simulink model "hybridSysSim"  (R2014b)
settings: Solver=ode45  SolverMode=SingleTasking  StartTime=0.0  StopTime=5  RelTol=1e-3
(part 1 of 2)
settings Model: Creator=Ricardo  LastModifiedBy=ricardog
settings OptimizationCC: BlockReduction=off  BooleanDataType=off
settings DebuggingCC: SaveWithParameterizedLinksMsg=none  UnderspecifiedInitializationDetection=Classic  MergeDetectMultiDrivingBlocksExec=none  SignalResolutionControl=TryResolveAllWithWarning  SolverPrmCheckMsg=none
settings HardwareCC: TargetUnknown=on

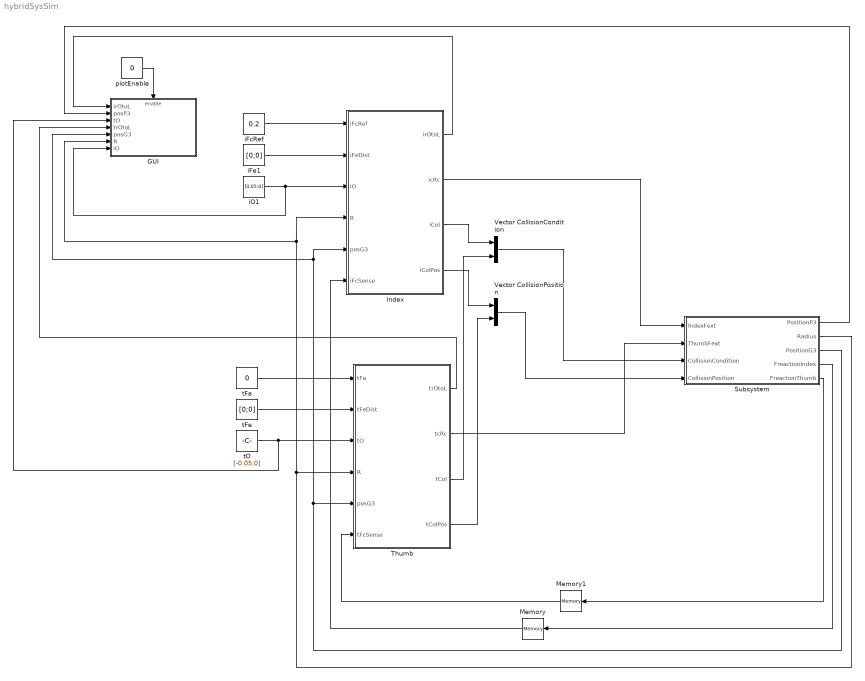
== system hybridSysSim ==
  GUI : Subsystem  TreatAsAtomicUnit=on
  Index : Subsystem
  Memory : Memory  InheritSampleTime=on
  Memory1 : Memory  InheritSampleTime=on
  Subsystem : Subsystem
  Thumb : Subsystem
  Vector CollisionCondition : Concatenate  Mode=Multidimensional array  ConcatenateDimension=2
  Vector CollisionPosition : Concatenate  Mode=Multidimensional array  ConcatenateDimension=2
  iFcRef : Constant  Value=0.2
  iFe1 : Constant  Value=[0;0]
  iO1 : Constant  Value=[0.05;0]
  plotEnable : Constant  Value=0
  tFa : Constant  Value=0
  tFe : Constant  Value=[0;0]
  tO : Constant  Value=[-0.05;0]
  wires:
  Thumb/2(tcRc) -> Subsystem/2(ThumbFext)
  plotEnable/1 -> GUI/Enable
  iFcRef/1 -> Index/1(iFcRef)
  iFe1/1 -> Index/2(iFeDist)
  iO1/1 -> GUI/7(iO), Index/3(iO)
  Index/3(iCol) -> Vector CollisionCondition/1
  Vector CollisionCondition/1 -> Subsystem/3(CollisionCondition)
  Vector CollisionPosition/1 -> Subsystem/4(CollisionPosition)
  Index/2(icRc) -> Subsystem/1(IndexFext)
  Subsystem/3(PositionG3) -> Thumb/5(posG3), GUI/5(posG3), Index/5(posG3)
  Subsystem/2(Radius) -> Thumb/4(R), GUI/6(R), Index/4(R)
  Subsystem/4(FreactionIndex) -> Memory/1
  Memory/1 -> Index/6(iFcSense)
  Index/4(iColPos) -> Vector CollisionPosition/1
  Index/1(irOtoL) -> GUI/1(irOtoL)
  Subsystem/1(PositionP3) -> GUI/2(posP3)
  Thumb/4(tColPos) -> Vector CollisionPosition/2
  Thumb/3(tCol) -> Vector CollisionCondition/2
  tFe/1 -> Thumb/2(tFeDist)
  tFa/1 -> Thumb/1(tFa)
  Memory1/1 -> Thumb/6(tFcSense)
  Subsystem/5(FreactionThumb) -> Memory1/1
  Thumb/1(trOtoL) -> GUI/4(trOtoL)
  tO/1 -> GUI/3(tO), Thumb/3(tO)

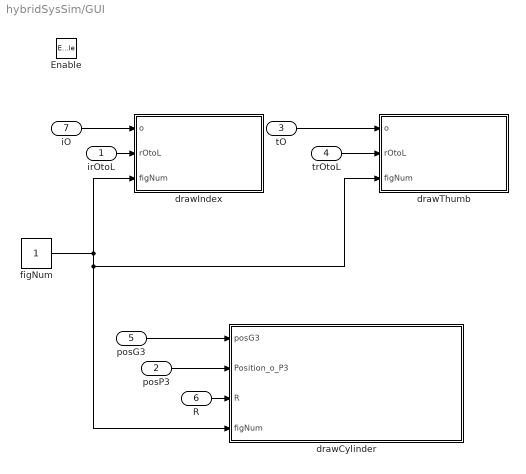
== system hybridSysSim/GUI ==
  irOtoL : Inport
  posP3 : Inport  Port=2
  tO : Inport  Port=3
  trOtoL : Inport  Port=4
  posG3 : Inport  Port=5
  R : Inport  Port=6
  iO : Inport  Port=7
  Enable : EnablePort
  drawCylinder : MATLAB Function  TreatAsAtomicUnit=on
  drawIndex : MATLAB Function  TreatAsAtomicUnit=on
  drawThumb : MATLAB Function  TreatAsAtomicUnit=on
  figNum : Constant
  wires:
  figNum/1 -> drawThumb/3(figNum), drawCylinder/4(figNum), drawIndex/3(figNum)
  posG3/1 -> drawCylinder/1(posG3)
  posP3/1 -> drawCylinder/2(Position_o_P3)
  irOtoL/1 -> drawIndex/2(rOtoL)
  iO/1 -> drawIndex/1(o)
  R/1 -> drawCylinder/3(R)
  tO/1 -> drawThumb/1(o)
  trOtoL/1 -> drawThumb/2(rOtoL)

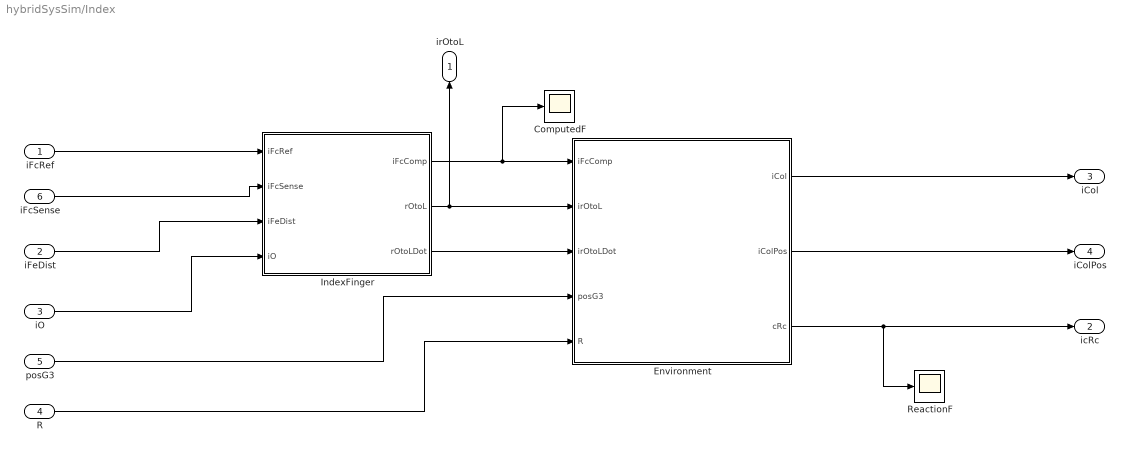
== system hybridSysSim/Index ==
  iFcRef : Inport
  iFeDist : Inport  Port=2
  iO : Inport  Port=3
  R : Inport  Port=4
  posG3 : Inport  Port=5
  iFcSense : Inport  Port=6
  ComputedF : Scope
      settings: YMin=-1.58123  YMax=0.18792
  Environment : Subsystem
  IndexFinger : Subsystem
  ReactionF : Scope
      settings: YMin=-2.47005  YMax=0.87632  SaveName=ScopeData2
  irOtoL : Outport
  icRc : Outport  Port=2
  iCol : Outport  Port=3
  iColPos : Outport  Port=4
  wires:
  IndexFinger/1(iFcComp) -> ComputedF/1, Environment/1(iFcComp)
  IndexFinger/2(rOtoL) -> irOtoL/1, Environment/2(irOtoL)
  IndexFinger/3(rOtoLDot) -> Environment/3(irOtoLDot)
  iFcRef/1 -> IndexFinger/1(iFcRef)
  iFcSense/1 -> IndexFinger/2(iFcSense)
  iFeDist/1 -> IndexFinger/3(iFeDist)
  iO/1 -> IndexFinger/4(iO)
  posG3/1 -> Environment/4(posG3)
  R/1 -> Environment/5(R)
  Environment/1(iCol) -> iCol/1
  Environment/2(iColPos) -> iColPos/1
  Environment/3(cRc) -> ReactionF/1, icRc/1

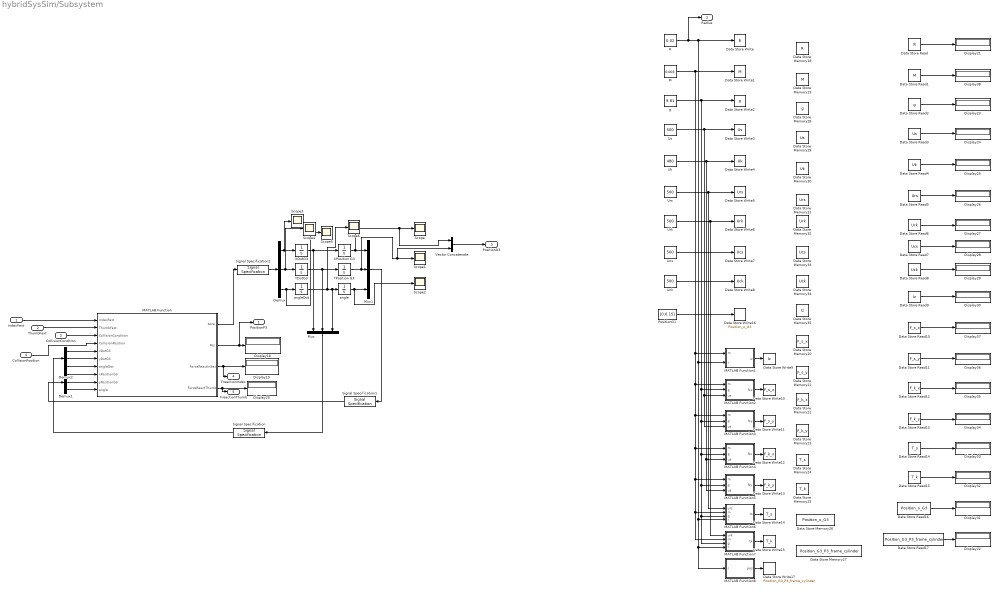
== system hybridSysSim/Subsystem ==
  IndexFext : Inport
  ThumbFext : Inport  Port=2
  CollisionCondition : Inport  Port=3
  CollisionPosition : Inport  Port=4
  Data Store Memory18 : DataStoreMemory  DataStoreName=R  ReadBeforeWriteMsg=warning  WriteAfterWriteMsg=warning  WriteAfterReadMsg=warning  OutDataTypeStr=double
  Data Store Memory19 : DataStoreMemory  DataStoreName=M  ReadBeforeWriteMsg=warning  WriteAfterWriteMsg=warning  WriteAfterReadMsg=warning  InitialValue=0.003  OutDataTypeStr=double
  Data Store Memory20 : DataStoreMemory  DataStoreName=F_s_x  ReadBeforeWriteMsg=warning  WriteAfterWriteMsg=warning  WriteAfterReadMsg=warning  OutDataTypeStr=double
  Data Store Memory21 : DataStoreMemory  DataStoreName=F_s_y  ReadBeforeWriteMsg=warning  WriteAfterWriteMsg=warning  WriteAfterReadMsg=warning  OutDataTypeStr=double
  Data Store Memory22 : DataStoreMemory  DataStoreName=F_k_x  ReadBeforeWriteMsg=warning  WriteAfterWriteMsg=warning  WriteAfterReadMsg=warning  OutDataTypeStr=double
  Data Store Memory23 : DataStoreMemory  DataStoreName=F_k_y  ReadBeforeWriteMsg=warning  WriteAfterWriteMsg=warning  WriteAfterReadMsg=warning  OutDataTypeStr=double
  Data Store Memory24 : DataStoreMemory  DataStoreName=T_s  ReadBeforeWriteMsg=warning  WriteAfterWriteMsg=warning  WriteAfterReadMsg=warning  OutDataTypeStr=double
  Data Store Memory25 : DataStoreMemory  DataStoreName=T_k  ReadBeforeWriteMsg=warning  WriteAfterWriteMsg=warning  WriteAfterReadMsg=warning  OutDataTypeStr=double
  Data Store Memory26 : DataStoreMemory  DataStoreName=Position_o_G3  ReadBeforeWriteMsg=warning  WriteAfterWriteMsg=warning  WriteAfterReadMsg=warning  InitialValue=[0;0]  OutDataTypeStr=double
  Data Store Memory27 : DataStoreMemory  DataStoreName=Position_G3_P3_frame_cylinder  ReadBeforeWriteMsg=warning  WriteAfterWriteMsg=warning  WriteAfterReadMsg=warning  InitialValue=[0;0]  OutDataTypeStr=double
  Data Store Memory28 : DataStoreMemory  DataStoreName=g  ReadBeforeWriteMsg=warning  WriteAfterWriteMsg=warning  WriteAfterReadMsg=warning  InitialValue=9.81  OutDataTypeStr=double
  Data Store Memory29 : DataStoreMemory  DataStoreName=Us  ReadBeforeWriteMsg=warning  WriteAfterWriteMsg=warning  WriteAfterReadMsg=warning  InitialValue=0.5  OutDataTypeStr=double
  Data Store Memory30 : DataStoreMemory  DataStoreName=Uk  ReadBeforeWriteMsg=warning  WriteAfterWriteMsg=warning  WriteAfterReadMsg=warning  InitialValue=0.48  OutDataTypeStr=double
  Data Store Memory31 : DataStoreMemory  DataStoreName=Urs  ReadBeforeWriteMsg=warning  WriteAfterWriteMsg=warning  WriteAfterReadMsg=warning  InitialValue=0.5  OutDataTypeStr=double
  Data Store Memory32 : DataStoreMemory  DataStoreName=Urk  ReadBeforeWriteMsg=warning  WriteAfterWriteMsg=warning  WriteAfterReadMsg=warning  InitialValue=0.48  OutDataTypeStr=double
  Data Store Memory33 : DataStoreMemory  DataStoreName=Ucs  ReadBeforeWriteMsg=warning  WriteAfterWriteMsg=warning  WriteAfterReadMsg=warning  InitialValue=0.5  OutDataTypeStr=double
  Data Store Memory34 : DataStoreMemory  DataStoreName=Uck  ReadBeforeWriteMsg=warning  WriteAfterWriteMsg=warning  WriteAfterReadMsg=warning  InitialValue=0.4  OutDataTypeStr=double
  Data Store Memory35 : DataStoreMemory  DataStoreName=Iz  ReadBeforeWriteMsg=warning  WriteAfterWriteMsg=warning  WriteAfterReadMsg=warning  OutDataTypeStr=double
  Data Store Read : DataStoreRead  DataStoreName=R
  Data Store Read1 : DataStoreRead  DataStoreName=M
  Data Store Read10 : DataStoreRead  DataStoreName=F_s_x
  Data Store Read11 : DataStoreRead  DataStoreName=F_s_y
  Data Store Read12 : DataStoreRead  DataStoreName=F_k_x
  Data Store Read13 : DataStoreRead  DataStoreName=F_k_y
  Data Store Read14 : DataStoreRead  DataStoreName=T_s
  Data Store Read15 : DataStoreRead  DataStoreName=T_k
  Data Store Read16 : DataStoreRead  DataStoreName=Position_o_G3
  Data Store Read17 : DataStoreRead  DataStoreName=Position_G3_P3_frame_cylinder
  Data Store Read2 : DataStoreRead  DataStoreName=g
  Data Store Read3 : DataStoreRead  DataStoreName=Us
  Data Store Read4 : DataStoreRead  DataStoreName=Uk
  Data Store Read5 : DataStoreRead  DataStoreName=Urs
  Data Store Read6 : DataStoreRead  DataStoreName=Urk
  Data Store Read7 : DataStoreRead  DataStoreName=Ucs
  Data Store Read8 : DataStoreRead  DataStoreName=Uck
  Data Store Read9 : DataStoreRead  DataStoreName=Iz
  Data Store Write : DataStoreWrite  DataStoreName=R
  Data Store Write1 : DataStoreWrite  DataStoreName=M
  Data Store Write10 : DataStoreWrite  DataStoreName=F_s_x
  Data Store Write11 : DataStoreWrite  DataStoreName=F_s_y
  Data Store Write12 : DataStoreWrite  DataStoreName=F_k_x
  Data Store Write13 : DataStoreWrite  DataStoreName=F_k_y
  Data Store Write14 : DataStoreWrite  DataStoreName=T_s
  Data Store Write15 : DataStoreWrite  DataStoreName=T_k
  Data Store Write16 : DataStoreWrite  DataStoreName=Position_o_G3
  Data Store Write17 : DataStoreWrite  DataStoreName=Position_G3_P3_frame_cylinder
  Data Store Write2 : DataStoreWrite  DataStoreName=g
  Data Store Write3 : DataStoreWrite  DataStoreName=Us
  Data Store Write4 : DataStoreWrite  DataStoreName=Uk
  Data Store Write5 : DataStoreWrite  DataStoreName=Urs
  Data Store Write6 : DataStoreWrite  DataStoreName=Urk
  Data Store Write7 : DataStoreWrite  DataStoreName=Ucs
  Data Store Write8 : DataStoreWrite  DataStoreName=Uck
  Data Store Write9 : DataStoreWrite  DataStoreName=Iz
  Demux : Demux  Outputs=3
  Demux1 : Demux  Outputs=3
  Demux2 : Demux  Outputs=3
  Display{18..38} (21 alike) : Display
  M : Constant  Value=0.003
  MATLAB Function : MATLAB Function  TreatAsAtomicUnit=on
  MATLAB Function1 : MATLAB Function  TreatAsAtomicUnit=on
  MATLAB Function2 : MATLAB Function  TreatAsAtomicUnit=on
  MATLAB Function3 : MATLAB Function  TreatAsAtomicUnit=on
  MATLAB Function4 : MATLAB Function  TreatAsAtomicUnit=on
  MATLAB Function5 : MATLAB Function  TreatAsAtomicUnit=on
  MATLAB Function6 : MATLAB Function  TreatAsAtomicUnit=on
  MATLAB Function7 : MATLAB Function  TreatAsAtomicUnit=on
  MATLAB Function8 : MATLAB Function  TreatAsAtomicUnit=on
  Mux : Mux  Inputs=3
  Mux1 : Mux  Inputs=3
  PositionG1 : Constant  Value=[0;0.15]
  R : Constant  Value=0.02
  Scope{,1..6} (7 alike) : Scope
  Signal Specification : SignalSpecification  Dimensions=3
  Signal Specification1 : SignalSpecification  Dimensions=3
  Signal Specification2 : SignalSpecification  Dimensions=3
  Uck : Constant  Value=500
  Ucs : Constant  Value=500
  Uk : Constant  Value=480
  Urk : Constant  Value=500
  Urs : Constant  Value=500
  Us : Constant  Value=500
  Vector Concatenate : Concatenate
  XDotG3 : Integrator
  XPosition G3 : Integrator
  YDotG3 : Integrator
  YPosition G3 : Integrator  InitialCondition=0.15
  angle : Integrator
  angleDot : Integrator
  g : Constant  Value=9.81
  PositionP3 : Outport
  Radius : Outport  Port=2
  PositionG3 : Outport  Port=3
  FreactionIndex : Outport  Port=4
  FreactionThumb : Outport  Port=5
  wires:
  MATLAB Function/1(Acce) -> Signal Specification2/1
  Demux/1 -> Scope3/1, XDotG3/1
  Demux/2 -> Scope4/1, YDotG3/1
  Demux/3 -> Scope5/1, angleDot/1
  XDotG3/1 -> Mux/1, XPosition G3/1
  YDotG3/1 -> Mux/2, YPosition G3/1
  angleDot/1 -> Scope6/1, Mux/3, angle/1
  XPosition G3/1 -> Vector Concatenate/1, Scope/1, Mux1/1
  angle/1 -> Scope2/1, Mux1/3
  YPosition G3/1 -> Vector Concatenate/2, Scope1/1, Mux1/2
  Mux1/1 -> Signal Specification1/1
  Mux/1 -> Signal Specification/1
  Signal Specification1/1 -> Demux1/1
  Demux1/1 -> MATLAB Function/8(xPositionG3)
  Demux1/2 -> MATLAB Function/9(yPositionG3)
  Demux1/3 -> MATLAB Function/10(angle)
  Signal Specification/1 -> Demux2/1
  Demux2/1 -> MATLAB Function/5(xDotG3)
  Demux2/2 -> MATLAB Function/6(yDotG3)
  Demux2/3 -> MATLAB Function/7(angleDot)
  IndexFext/1 -> MATLAB Function/1(IndexFext)
  ThumbFext/1 -> MATLAB Function/2(ThumbFext)
  CollisionCondition/1 -> MATLAB Function/3(CollisionCondition)
  CollisionPosition/1 -> MATLAB Function/4(CollisionPosition)
  Signal Specification2/1 -> Demux/1
  MATLAB Function/2(Pos) -> PositionP3/1, Display18/1
  MATLAB Function/3(ForceReactIndex) -> FreactionIndex/1, Display19/1
  MATLAB Function/4(ForceReactThumb) -> FreactionThumb/1, Display20/1
  R/1 -> Radius/1, MATLAB Function6/4(r), MATLAB Function7/4(r), MATLAB Function8/1(r), MATLAB Function1/2(r), Data Store Write/1
  M/1 -> MATLAB Function1/1(m), MATLAB Function2/1(m), MATLAB Function3/1(m), MATLAB Function4/1(m), MATLAB Function5/1(m), MATLAB Function6/2(m), MATLAB Function7/2(m), Data Store Write1/1
  g/1 -> Data Store Write2/1, MATLAB Function2/2(g), MATLAB Function3/2(g), MATLAB Function4/2(g), MATLAB Function5/2(g), MATLAB Function6/3(g), MATLAB Function7/3(g)
  Us/1 -> Data Store Write3/1, MATLAB Function2/3(us), MATLAB Function3/3(us)
  Uk/1 -> MATLAB Function4/3(uk), MATLAB Function5/3(uk), Data Store Write4/1
  Urs/1 -> MATLAB Function6/1(urs), Data Store Write5/1
  Urk/1 -> MATLAB Function7/1(urk), Data Store Write6/1
  Ucs/1 -> Data Store Write7/1
  Uck/1 -> Data Store Write8/1
  Data Store Read/1 -> Display21/1
  Data Store Read1/1 -> Display38/1
  Data Store Read2/1 -> Display23/1
  Data Store Read3/1 -> Display24/1
  Data Store Read4/1 -> Display25/1
  Data Store Read5/1 -> Display26/1
  Data Store Read6/1 -> Display27/1
  Data Store Read7/1 -> Display28/1
  Data Store Read8/1 -> Display29/1
  Data Store Read9/1 -> Display30/1
  Data Store Read10/1 -> Display37/1
  Data Store Read11/1 -> Display36/1
  Data Store Read12/1 -> Display35/1
  Data Store Read13/1 -> Display34/1
  Data Store Read14/1 -> Display33/1
  Data Store Read15/1 -> Display32/1
  Data Store Read16/1 -> Display31/1
  Data Store Read17/1 -> Display22/1
  MATLAB Function1/1(iz) -> Data Store Write9/1
  MATLAB Function2/1(fsx) -> Data Store Write10/1
  MATLAB Function3/1(fsy) -> Data Store Write11/1
  MATLAB Function4/1(fkx) -> Data Store Write12/1
  MATLAB Function5/1(fky) -> Data Store Write13/1
  MATLAB Function6/1(ts) -> Data Store Write14/1
  MATLAB Function7/1(tk) -> Data Store Write15/1
  MATLAB Function8/1(pos) -> Data Store Write17/1
  PositionG1/1 -> Data Store Write16/1
  Vector Concatenate/1 -> PositionG3/1

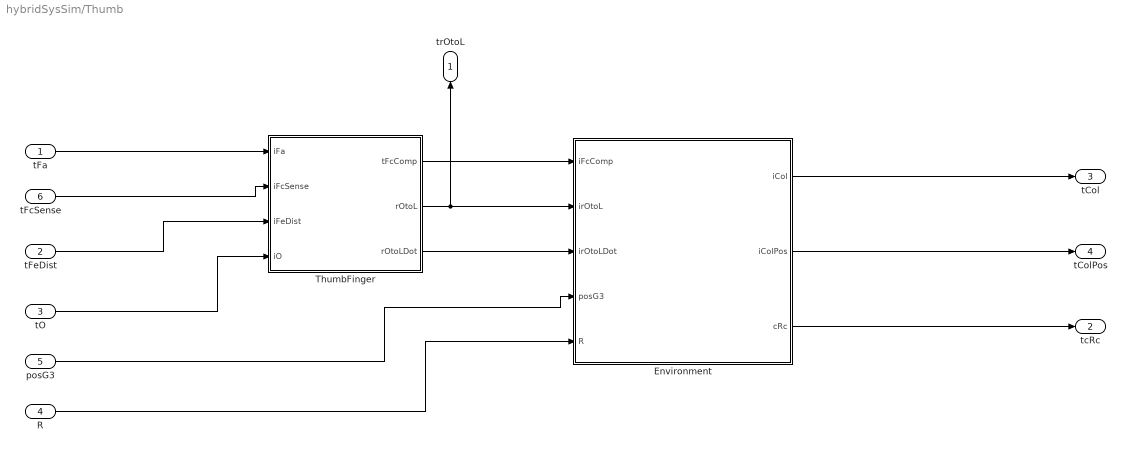
== system hybridSysSim/Thumb ==
  tFa : Inport
  tFeDist : Inport  Port=2
  tO : Inport  Port=3
  R : Inport  Port=4
  posG3 : Inport  Port=5
  tFcSense : Inport  Port=6
  Environment : Subsystem
  ThumbFinger : Subsystem
  trOtoL : Outport
  tcRc : Outport  Port=2
  tCol : Outport  Port=3
  tColPos : Outport  Port=4
  wires:
  ThumbFinger/1(tFcComp) -> Environment/1(iFcComp)
  ThumbFinger/2(rOtoL) -> trOtoL/1, Environment/2(irOtoL)
  ThumbFinger/3(rOtoLDot) -> Environment/3(irOtoLDot)
  tFa/1 -> ThumbFinger/1(iFa)
  tFcSense/1 -> ThumbFinger/2(iFcSense)
  tFeDist/1 -> ThumbFinger/3(iFeDist)
  tO/1 -> ThumbFinger/4(iO)
  posG3/1 -> Environment/4(posG3)
  R/1 -> Environment/5(R)
  Environment/1(iCol) -> tCol/1
  Environment/2(iColPos) -> tColPos/1
  Environment/3(cRc) -> tcRc/1

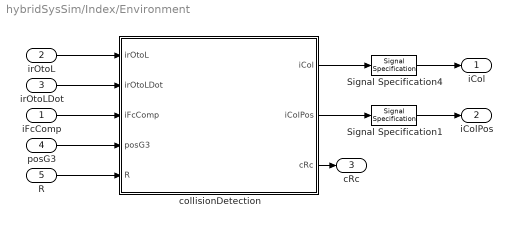
== system hybridSysSim/Index/Environment ==
  iFcComp : Inport
  irOtoL : Inport  Port=2
  irOtoLDot : Inport  Port=3
  posG3 : Inport  Port=4
  R : Inport  Port=5
  Signal Specification1 : SignalSpecification  Dimensions=2
  Signal Specification4 : SignalSpecification  Dimensions=1
  collisionDetection : MATLAB Function  TreatAsAtomicUnit=on
  iCol : Outport
  iColPos : Outport  Port=2
  cRc : Outport  Port=3
  wires:
  irOtoLDot/1 -> collisionDetection/2(irOtoLDot)
  irOtoL/1 -> collisionDetection/1(irOtoL)
  posG3/1 -> collisionDetection/4(posG3)
  collisionDetection/1(iCol) -> Signal Specification4/1
  collisionDetection/2(iColPos) -> Signal Specification1/1
  R/1 -> collisionDetection/5(R)
  collisionDetection/3(cRc) -> cRc/1
  iFcComp/1 -> collisionDetection/3(iFcComp)
  Signal Specification4/1 -> iCol/1
  Signal Specification1/1 -> iColPos/1

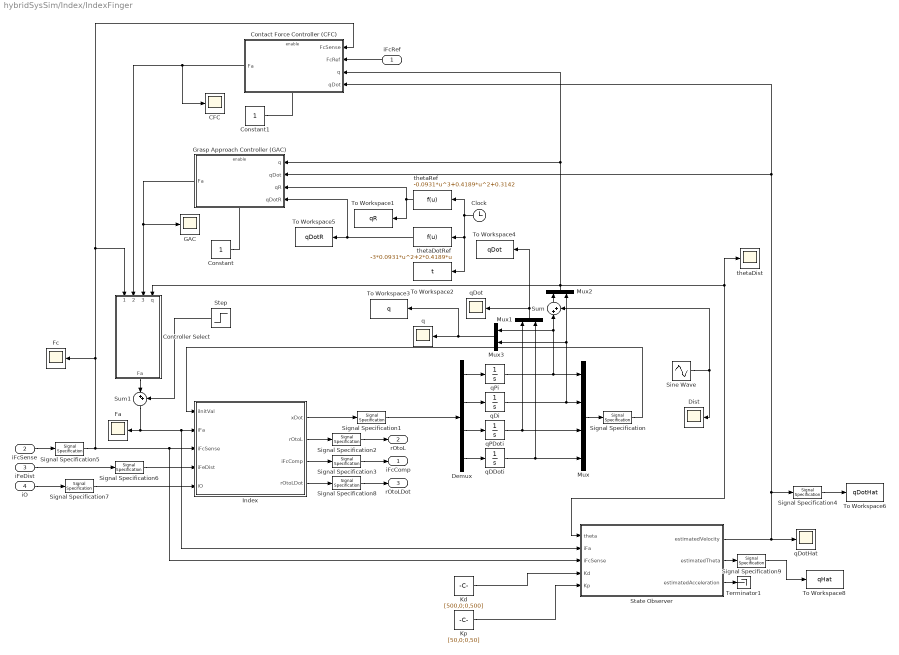
== system hybridSysSim/Index/IndexFinger ==
  iFcRef : Inport
  iFcSense : Inport  Port=2
  iFeDist : Inport  Port=3
  iO : Inport  Port=4
  CFC : Scope
      settings: YMin=-0.35871  YMax=5.16957
  Clock : Clock
  Constant : Constant
  Constant1 : Constant
  Contact Force Controller (CFC) : Subsystem  TreatAsAtomicUnit=on
  Controller Select : MATLAB Function  TreatAsAtomicUnit=on
  Demux : Demux
  Dist : Scope
      settings: YMin=-1.00000  YMax=1.00000  SaveName=ScopeData2
  Fa : Scope
      settings: YMin=-117.77847  YMax=155.15586  SaveName=ScopeData4
  Fc : Scope
      settings: YMin=-0.25995  YMax=0.60021  SaveName=ScopeData3
  GAC : Scope
      settings: YMin=-5.60577  YMax=50.52435  SaveName=ScopeData2
  Grasp Approach Controller (GAC) : Subsystem  TreatAsAtomicUnit=on
  Index : MATLAB Function  TreatAsAtomicUnit=on
  Kd : Constant  Value=[500,0;0,500]
  Kp : Constant  Value=[50,0;0,50]
  Mux : Mux
  Mux1 : Mux  Inputs=2
  Mux2 : Mux  Inputs=2
  Mux3 : Mux  Inputs=2
  Signal Specification : SignalSpecification  Dimensions=4
  Signal Specification1 : SignalSpecification  Dimensions=4
  Signal Specification2 : SignalSpecification  Dimensions=[2 2]
  Signal Specification{3,5..8} (5 alike) : SignalSpecification  Dimensions=[2 1]
  Signal Specification4 : SignalSpecification  Dimensions=2
  Signal Specification9 : SignalSpecification  Dimensions=2
  Sine Wave : Sin  Amplitude=0  Frequency=5000  SampleTime=0
  State Observer : Subsystem
  Step : Step  After=0  SampleTime=0
  Sum : Sum  Inputs=|++
  Sum1 : Sum  Inputs=|++
  Terminator1 : Terminator
  To Workspace1 : ToWorkspace  VariableName=qR  SampleTime=-1
  To Workspace2 : ToWorkspace  VariableName=t  SampleTime=-1
  To Workspace3 : ToWorkspace  VariableName=q  SampleTime=-1
  To Workspace4 : ToWorkspace  VariableName=qDot  SampleTime=-1
  To Workspace5 : ToWorkspace  VariableName=qDotR  SampleTime=-1
  To Workspace6 : ToWorkspace  VariableName=qDotHat  SampleTime=-1
  To Workspace8 : ToWorkspace  VariableName=qHat  SampleTime=-1
  q : Scope
      settings: YMin=0.20609  YMax=1.28677  SaveName=ScopeData2
  qDDoti : Integrator  ContinuousStateAttributes='indexDistThetaDot'
  qDi : Integrator  InitialCondition=pi/3  ContinuousStateAttributes='indexDistTheta'
  qDot : Scope
      settings: YMin=-1.79916  YMax=2.42907
  qDotHat : Scope
      settings: YMin=-26.19585  YMax=32.38783  SaveName=ScopeData3
  qPDoti : Integrator  ContinuousStateAttributes='indexProxThetaDot'
  qPi : Integrator  InitialCondition=pi/10  ContinuousStateAttributes='indexProxTheta'
  thetaDist : Scope
      settings: YMin=0.18138  YMax=1.5092
  thetaDotRef : Fcn  Expr=-3*0.0931*u^2+2*0.4189*u
  thetaRef : Fcn  Expr=-0.0931*u^3+0.4189*u^2+0.3142
  iFcComp : Outport
  rOtoL : Outport  Port=2
  rOtoLDot : Outport  Port=3
  wires:
  Demux/1 -> qPi/1
  Demux/2 -> qDi/1
  Demux/3 -> qPDoti/1
  Demux/4 -> qDDoti/1
  qPi/1 -> Mux3/1, Sum/1, Mux/1
  qDi/1 -> Mux2/2, Mux3/2, Mux/2
  qPDoti/1 -> Mux1/1, Mux/3
  qDDoti/1 -> Mux1/2, Mux/4
  Index/1(xDot) -> Signal Specification1/1
  Mux/1 -> Signal Specification/1
  Index/2(rOtoL) -> Signal Specification2/1
  Signal Specification/1 -> Index/1(iInitVal)
  Signal Specification1/1 -> Demux/1
  iFcSense/1 -> Signal Specification5/1
  iFeDist/1 -> Signal Specification6/1
  iO/1 -> Signal Specification7/1
  Signal Specification2/1 -> rOtoL/1
  Signal Specification3/1 -> iFcComp/1
  Index/3(iFcComp) -> Signal Specification3/1
  Signal Specification6/1 -> Index/4(iFeDist)
  Signal Specification7/1 -> Index/5(iO)
  Signal Specification8/1 -> rOtoLDot/1
  Index/4(rOtoLDot) -> Signal Specification8/1
  Contact Force Controller (CFC)/1(Fa) -> Controller Select/2(CFC), CFC/1
  Grasp Approach Controller (GAC)/1(Fa) -> GAC/1, Controller Select/3(GAC)
  iFcRef/1 -> Contact Force Controller (CFC)/2(FcRef)
  thetaRef/1 -> Grasp Approach Controller (GAC)/3(qR), To Workspace1/1
  Clock/1 -> To Workspace2/1, thetaDotRef/1, thetaRef/1
  thetaDotRef/1 -> To Workspace5/1, Grasp Approach Controller (GAC)/4(qDotR)
  Constant1/1 -> Contact Force Controller (CFC)/Enable
  Constant/1 -> Grasp Approach Controller (GAC)/Enable
  Signal Specification5/1 -> State Observer/3(iFcSense), Index/3(iFcSense), Fc/1, Controller Select/1(FcSense), Contact Force Controller (CFC)/1(FcSense)
  Kd/1 -> State Observer/4(Kd)
  Kp/1 -> State Observer/5(Kp)
  State Observer/2(estimatedTheta) -> Signal Specification9/1
  State Observer/3(estimatedAcceleration) -> Terminator1/1
  Signal Specification4/1 -> To Workspace6/1
  State Observer/1(estimatedVelocity) -> Contact Force Controller (CFC)/4(qDot), Grasp Approach Controller (GAC)/2(qDot), Signal Specification4/1, qDotHat/1
  Mux1/1 -> To Workspace4/1, qDot/1
  Sine Wave/1 -> Dist/1, Sum/2
  Controller Select/1(Fa) -> Sum1/1
  Sum1/1 -> Fa/1, State Observer/2(iFa), Index/2(iFa)
  Step/1 -> Sum1/2
  Sum/1 -> Mux2/1
  Mux2/1 -> State Observer/1(theta), thetaDist/1, Contact Force Controller (CFC)/3(q), Grasp Approach Controller (GAC)/1(q), Controller Select/4(q)
  Mux3/1 -> To Workspace3/1, q/1
  Signal Specification9/1 -> To Workspace8/1

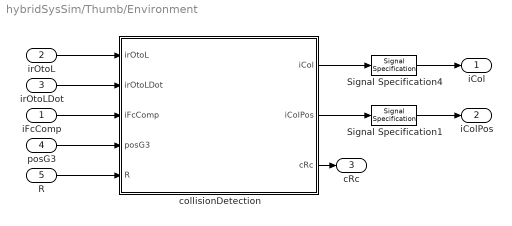
== system hybridSysSim/Thumb/Environment ==
  iFcComp : Inport
  irOtoL : Inport  Port=2
  irOtoLDot : Inport  Port=3
  posG3 : Inport  Port=4
  R : Inport  Port=5
  Signal Specification1 : SignalSpecification  Dimensions=2
  Signal Specification4 : SignalSpecification  Dimensions=1
  collisionDetection : MATLAB Function  TreatAsAtomicUnit=on
  iCol : Outport
  iColPos : Outport  Port=2
  cRc : Outport  Port=3
  wires:
  irOtoLDot/1 -> collisionDetection/2(irOtoLDot)
  irOtoL/1 -> collisionDetection/1(irOtoL)
  posG3/1 -> collisionDetection/4(posG3)
  collisionDetection/1(iCol) -> Signal Specification4/1
  collisionDetection/2(iColPos) -> Signal Specification1/1
  R/1 -> collisionDetection/5(R)
  collisionDetection/3(cRc) -> cRc/1
  iFcComp/1 -> collisionDetection/3(iFcComp)
  Signal Specification4/1 -> iCol/1
  Signal Specification1/1 -> iColPos/1

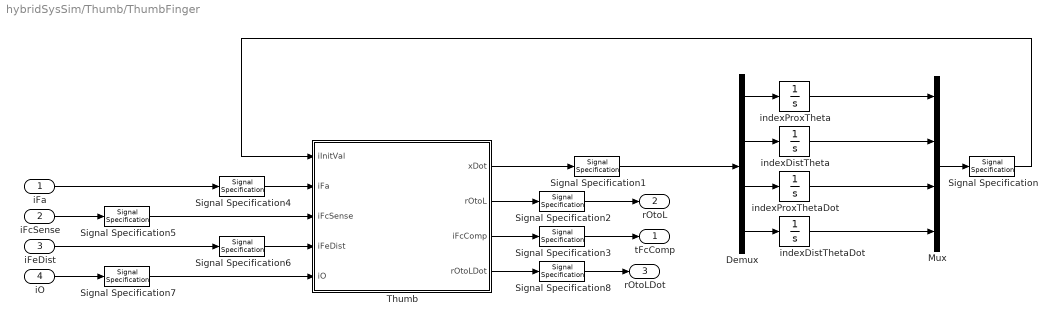
== system hybridSysSim/Thumb/ThumbFinger ==
  iFa : Inport
  iFcSense : Inport  Port=2
  iFeDist : Inport  Port=3
  iO : Inport  Port=4
  Demux : Demux
  Mux : Mux
  Signal Specification : SignalSpecification  Dimensions=4
  Signal Specification1 : SignalSpecification  Dimensions=4
  Signal Specification2 : SignalSpecification  Dimensions=[2 2]
  Signal Specification{3,5..8} (5 alike) : SignalSpecification  Dimensions=[2 1]
  Signal Specification4 : SignalSpecification  Dimensions=1
  Thumb : MATLAB Function  TreatAsAtomicUnit=on
  indexDistTheta : Integrator  InitialCondition=-pi/3  ContinuousStateAttributes='indexDistTheta'
  indexDistThetaDot : Integrator  ContinuousStateAttributes='indexDistThetaDot'
  indexProxTheta : Integrator  InitialCondition=pi-pi/10  ContinuousStateAttributes='indexProxTheta'
  indexProxThetaDot : Integrator  ContinuousStateAttributes='indexProxThetaDot'
  tFcComp : Outport
  rOtoL : Outport  Port=2
  rOtoLDot : Outport  Port=3
  wires:
  Demux/1 -> indexProxTheta/1
  Demux/2 -> indexDistTheta/1
  Demux/3 -> indexProxThetaDot/1
  Demux/4 -> indexDistThetaDot/1
  indexProxTheta/1 -> Mux/1
  indexDistTheta/1 -> Mux/2
  indexProxThetaDot/1 -> Mux/3
  indexDistThetaDot/1 -> Mux/4
  Thumb/1(xDot) -> Signal Specification1/1
  Mux/1 -> Signal Specification/1
  Thumb/2(rOtoL) -> Signal Specification2/1
  Signal Specification/1 -> Thumb/1(iInitVal)
  Signal Specification1/1 -> Demux/1
  iFa/1 -> Signal Specification4/1
  iFcSense/1 -> Signal Specification5/1
  iFeDist/1 -> Signal Specification6/1
  iO/1 -> Signal Specification7/1
  Signal Specification2/1 -> rOtoL/1
  Signal Specification3/1 -> tFcComp/1
  Thumb/3(iFcComp) -> Signal Specification3/1
  Signal Specification4/1 -> Thumb/2(iFa)
  Signal Specification5/1 -> Thumb/3(iFcSense)
  Signal Specification6/1 -> Thumb/4(iFeDist)
  Signal Specification7/1 -> Thumb/5(iO)
  Signal Specification8/1 -> rOtoLDot/1
  Thumb/4(rOtoLDot) -> Signal Specification8/1

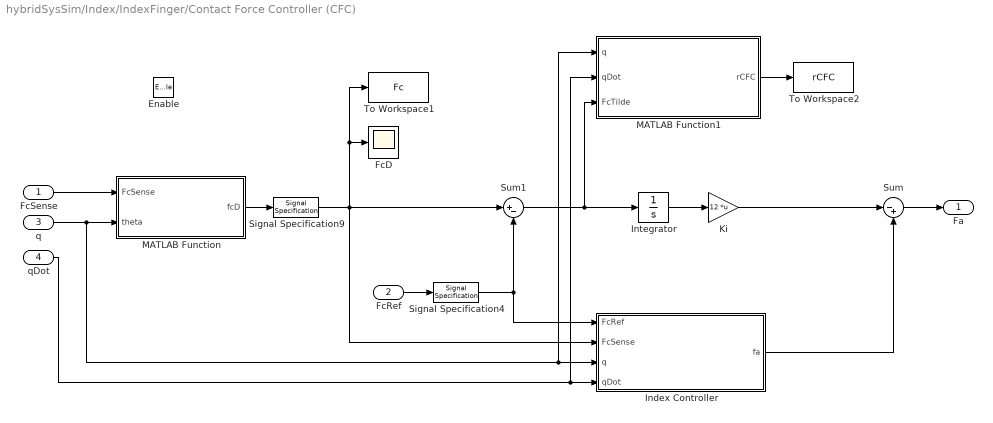
== system hybridSysSim/Index/IndexFinger/Contact Force Controller (CFC) ==
  FcSense : Inport
  FcRef : Inport  Port=2
  q : Inport  Port=3
  qDot : Inport  Port=4
  Enable : EnablePort  StatesWhenEnabling=reset
  FcD : Scope
      settings: YMin=-0.06018  YMax=0.54162  SaveName=ScopeData5
  Index Controller : MATLAB Function  TreatAsAtomicUnit=on
  Integrator : Integrator  ContinuousStateAttributes='ErrorIntegral'
  Ki : Gain  Gain=12  Multiplication=Matrix(K*u) (u vector)
  MATLAB Function : MATLAB Function  TreatAsAtomicUnit=on
  MATLAB Function1 : MATLAB Function  TreatAsAtomicUnit=on
  Signal Specification4 : SignalSpecification  Dimensions=1
  Signal Specification9 : SignalSpecification  Dimensions=1
  Sum : Sum  Inputs=|-+
  Sum1 : Sum  Inputs=|+-
  To Workspace1 : ToWorkspace  VariableName=Fc  SampleTime=-1
  To Workspace2 : ToWorkspace  VariableName=rCFC  SampleTime=-1
  Fa : Outport
  wires:
  FcRef/1 -> Signal Specification4/1
  Signal Specification4/1 -> Index Controller/1(FcRef), Sum1/2
  FcSense/1 -> MATLAB Function/1(FcSense)
  Sum/1 -> Fa/1
  Sum1/1 -> MATLAB Function1/3(FcTilde), Integrator/1
  Integrator/1 -> Ki/1
  Ki/1 -> Sum/1
  MATLAB Function/1(fcD) -> Signal Specification9/1
  Signal Specification9/1 -> FcD/1, To Workspace1/1, Sum1/1, Index Controller/2(FcSense)
  qDot/1 -> MATLAB Function1/2(qDot), Index Controller/4(qDot)
  q/1 -> MATLAB Function/2(theta), MATLAB Function1/1(q), Index Controller/3(q)
  Index Controller/1(fa) -> Sum/2
  MATLAB Function1/1(rCFC) -> To Workspace2/1

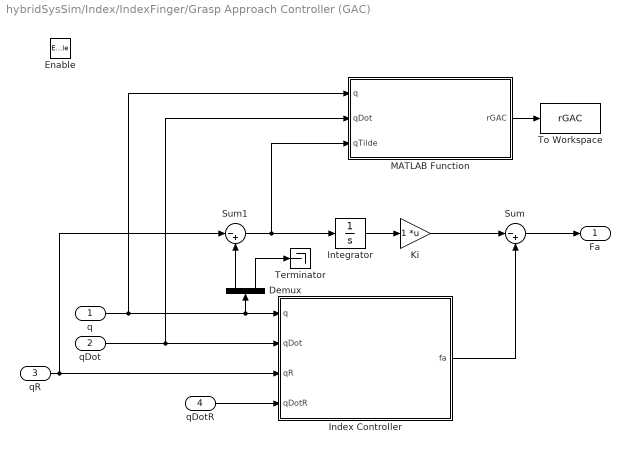
== system hybridSysSim/Index/IndexFinger/Grasp Approach Controller (GAC) ==
  q : Inport
  qDot : Inport  Port=2
  qR : Inport  Port=3
  qDotR : Inport  Port=4
  Enable : EnablePort  StatesWhenEnabling=reset
  Demux : Demux  Outputs=2
  Index Controller : MATLAB Function  TreatAsAtomicUnit=on
  Integrator : Integrator  ContinuousStateAttributes='ErrorIntegral'
  Ki : Gain  Multiplication=Matrix(K*u) (u vector)
  MATLAB Function : MATLAB Function  TreatAsAtomicUnit=on
  Sum : Sum  Inputs=|-+
  Sum1 : Sum  Inputs=|-+
  Terminator : Terminator
  To Workspace : ToWorkspace  VariableName=rGAC  SampleTime=-1
  Fa : Outport
  wires:
  q/1 -> MATLAB Function/1(q), Demux/1, Index Controller/1(q)
  qR/1 -> Index Controller/3(qR), Sum1/1
  qDotR/1 -> Index Controller/4(qDotR)
  Integrator/1 -> Ki/1
  Sum1/1 -> MATLAB Function/3(qTilde), Integrator/1
  Demux/1 -> Sum1/2
  Demux/2 -> Terminator/1
  Ki/1 -> Sum/1
  Index Controller/1(fa) -> Sum/2
  Sum/1 -> Fa/1
  qDot/1 -> MATLAB Function/2(qDot), Index Controller/2(qDot)
  MATLAB Function/1(rGAC) -> To Workspace/1

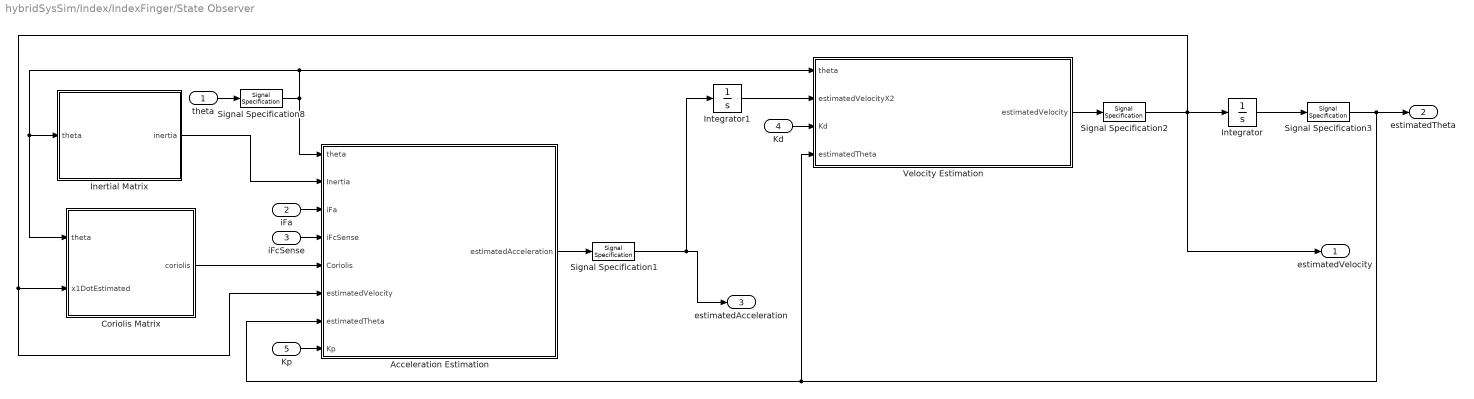
== system hybridSysSim/Index/IndexFinger/State Observer ==
  theta : Inport
  iFa : Inport  Port=2
  iFcSense : Inport  Port=3
  Kd : Inport  Port=4
  Kp : Inport  Port=5
  Acceleration Estimation : MATLAB Function  TreatAsAtomicUnit=on
  Coriolis Matrix : MATLAB Function  TreatAsAtomicUnit=on
  Inertial Matrix : MATLAB Function  TreatAsAtomicUnit=on
  Integrator : Integrator  InitialCondition=[pi/10;pi/3]  UpperSaturationLimit=1e100  LowerSaturationLimit=-1e100
  Integrator1 : Integrator  InitialCondition=[0;0]  UpperSaturationLimit=1e100  LowerSaturationLimit=-1e100
  Signal Specification{1..3,8} (4 alike) : SignalSpecification  Dimensions=[2 1]
  Velocity Estimation : MATLAB Function  TreatAsAtomicUnit=on
  estimatedVelocity : Outport
  estimatedTheta : Outport  Port=2
  estimatedAcceleration : Outport  Port=3
  wires:
  Inertial Matrix/1(inertia) -> Acceleration Estimation/2(Inertia)
  Coriolis Matrix/1(coriolis) -> Acceleration Estimation/5(Coriolis)
  Acceleration Estimation/1(estimatedAcceleration) -> Signal Specification1/1
  Velocity Estimation/1(estimatedVelocity) -> Signal Specification2/1
  theta/1 -> Signal Specification8/1
  iFa/1 -> Acceleration Estimation/3(iFa)
  iFcSense/1 -> Acceleration Estimation/4(iFcSense)
  Kd/1 -> Velocity Estimation/3(Kd)
  Kp/1 -> Acceleration Estimation/8(Kp)
  Integrator/1 -> Signal Specification3/1
  Integrator1/1 -> Velocity Estimation/2(estimatedVelocityX2)
  Signal Specification8/1 -> Acceleration Estimation/1(theta), Inertial Matrix/1(theta), Coriolis Matrix/1(theta), Velocity Estimation/1(theta)
  Signal Specification2/1 -> Integrator/1, Acceleration Estimation/6(estimatedVelocity), Coriolis Matrix/2(x1DotEstimated), estimatedVelocity/1
  Signal Specification3/1 -> Acceleration Estimation/7(estimatedTheta), Velocity Estimation/4(estimatedTheta), estimatedTheta/1
  Signal Specification1/1 -> Integrator1/1, estimatedAcceleration/1

== matlab function hybridSysSim/Subsystem/MATLAB Function ==
  data: IndexFext input; Acce output; ThumbFext input; CollisionCondition input; CollisionPosition input; xDotG3 input; yDotG3 input; angleDot input; xPositionG3 input; yPositionG3 input; angle input; Pos output; ForceReactIndex output; ForceReactThumb output; R data_store_memory; M data_store_memory; g data_store_memory; Us data_store_memory; Uk data_store_memory; Urs data_store_memory; Urk data_store_memory; Ucs data_store_memory; Uck data_store_memory; Iz data_store_memory; F_s_x data_store_memory; F_s_y data_store_memory; F_k_x data_store_memory; F_k_y data_store_memory; T_s data_store_memory; T_k data_store_memory; Position_o_G3 data_store_memory; Position_G3_P3_frame_cylinder data_store_memory
function [Acce,Pos,ForceReactIndex,ForceReactThumb] = CylinderMain(IndexFext,ThumbFext,CollisionCondition,...
                                                                   CollisionPosition,xDotG3,yDotG3,angleDot...
                                                                   ,xPositionG3,yPositionG3,angle)
%   global variables parameters
    global R M g Us Uk Urs Urk Ucs Uck Iz F_s_x F_s_y F_k_x F_k_y T_s T_k Position_o_G3 Position_G3_P3_frame_cylinder;
    R;%Radius of the cylindrical ect in meters
    M;%Mass of the ect in Kg
    g;%Acceleration of gravity in m/s^2
    Us;%Static coefficient of friction
    Uk;%Kinetic coefficient of friction
    Urs;%Static rotational coefficient of friction
    Urk;%Kinetic rotational coefficient of friction
    Ucs;%Static contact coefficient of friction
    Uck;%Kinetic contact coefficient of friction
    Iz;%Inertia of the cylindrical ect in Z
    F_s_x;%Static friction force in X
    F_s_y;%Static friction force in Y
    F_k_x;%Kinetic friction force in X
    F_k_y;%Kinetic friction force in Y
    T_s;%Static friction torque see derivation notes to verify the expression
    T_k;%Kinetic friction torque see derivation notes to verify the expression
    Position_o_G3;%Position from frame 0 to the centre of gravity of the cylinder
    Position_G3_P3_frame_cylinder;%Position to second point of the cylinder
    CollisionIndexForce=CollisionConditionFunct(CollisionCondition(1),IndexFext);
    CollisionThumbForce=CollisionConditionFunct(CollisionCondition(2),ThumbFext);
    GenCordExt=ForcesCalculator(CollisionIndexForce,CollisionThumbForce,CollisionPosition,xPositionG3,yPositionG3);
    GeneralCoordinatesDoubleDot = Equation_Of_Motion(GenCordExt);
    ForceReactionIndex=ForceReactionFinger(GeneralCoordinatesDoubleDot,CollisionIndexForce);
    ForceReactionThumb=ForceReactionFinger(GeneralCoordinatesDoubleDot,CollisionThumbForce);
    xDoubleDot = GeneralCoordinatesDoubleDot(1);
    yDoubleDot = GeneralCoordinatesDoubleDot(2);
    angleDoubleDot = GeneralCoordinatesDoubleDot(3);
    Positions = PosCalculation(angle,xPositionG3,yPositionG3);
    Velocities = VelCalculation (angle,angleDot,xDotG3,yDotG3);
    Accelerations = AccCalculation (angle,angleDot,angleDoubleDot,xDoubleDot,yDoubleDot);
    Acce=Accelerations([1 2 5]);
    Pos=Positions([3 4])';
    ForceReactIndex=ForceReactionIndex;
    ForceReactThumb=ForceReactionThumb;
end
    %............................................................................
    %............................................................................
    %Evaluates if the external force is greater than the static
    %friction forces or torques
function FrictionCondition=NonLinearFriction(GenCordExt,Election)
global F_s_x F_s_y T_s;
            %Evaluates wich static friction have to be compared
            if (strcmp(Election,'F_s_x')==1)
                ForceEvaluation=F_s_x;
            elseif(strcmp(Election,'F_s_y')==1)
                ForceEvaluation=F_s_y;
            else
                ForceEvaluation=T_s;
            end
            %Condition checker
            if(GenCordExt<=ForceEvaluation)
                FrictionCondition=0;%if the Friction condition is 0 there is no movement
            else
                FrictionCondition=1;%if the Friction condition is 1 there is movement
            end
end
    %............................................................................
    %............................................................................
    %Calculates the acceleration components in X and Y for the centre of
    %gravity of the ect and the angular acceleration
function GeneralCoordinatesDoubleDot = Equation_Of_Motion(GenCordExt)
global M Iz F_k_x F_k_y T_k ;
            GeneralCoordinatesDoubleDot=zeros(3);
            %Ecuation of motion for X coordinates
            SignOposite=-1*sign(GenCordExt);
            if(NonLinearFriction(abs(GenCordExt(1)),'F_s_x')== 1)
                GeneralCoordinatesDoubleDot(1)= (GenCordExt(1)+ SignOposite(1)*F_k_x)/M;
            else
                GeneralCoordinatesDoubleDot(1)= 0;
            end
        %Ecuation of motion for y coordinates
            if(NonLinearFriction(abs(GenCordExt(2)),'F_s_y')== 1)
                GeneralCoordinatesDoubleDot(2)= (GenCordExt(2)+ SignOposite(2)*F_k_y)/M;
            else
                GeneralCoordinatesDoubleDot(2)= 0;
            end
        %Ecuation of motion for Tetha coordinates
            if(NonLinearFriction(abs(GenCordExt(3)),'T_s')== 1)
                GeneralCoordinatesDoubleDot(3)= (GenCordExt(3)+ SignOposite(3)*T_k)/Iz;
            else
                GeneralCoordinatesDoubleDot(3)= 0;
            end
end
    %............................................................................
    %............................................................................
    %Absolute positions for G3 and P3 updated from frame 0
function Positions = PosCalculation(angle,xPositionG3,yPositionG3)
global Position_o_G3 Position_G3_P3_frame_cylinder;
            Rotation_o_3=[cos(angle),-sin(angle);sin(angle),cos(angle)];
            Position_G3_P3_frame_0=Rotation_o_3*Position_G3_P3_frame_cylinder;
            Position_o_P3=[xPositionG3;yPositionG3] + Position_G3_P3_frame_0;
            Positions=[Position_o_G3,Position_o_P3];
end
    %............................................................................
    %............................................................................
    %Absolute velocities for G3 and P3 updated from frame 0
function Velocities = VelCalculation (angle,angleDot,xDotG3,yDotG3)
global R;
            Velocity_o_G3_frame_0=[xDotG3;yDotG3];
            Velocity_o_P3_frame_0=[xDotG3-R*cos(angle)*angleDot;yDotG3-R*sin(angle)*angleDot];
            Velocities=[Velocity_o_G3_frame_0,Velocity_o_P3_frame_0];
end
    %............................................................................
    %............................................................................
    %Absolute Accelerations for G3 and P3 updated from frame 0
function Accelerations = AccCalculation (angle,angleDot,angleDoubleDot,xDoubleDot,yDoubleDot)
global R;
            Acceleration_o_G3_frame_0=[xDoubleDot;yDoubleDot];
            Acceleration_o_P3_frame_0=[xDoubleDot+R*sin(angle)*(angleDot^2)-R*cos(angle)*angleDoubleDot;...
                                       yDoubleDot-R*cos(angle)*(angleDot^2)-R*sin(angle)*angleDoubleDot];
            Accelerations=[Acceleration_o_G3_frame_0,Acceleration_o_P3_frame_0,[angleDoubleDot;0]];
end
    %............................................................................
    %............................................................................
    %Absolute Accelerations for G3 and P3 updated from frame 0
function RotMatrix_0_4=RotationToContactFrame(CollisionPosition,xPositionG3,yPositionG3)
            Theta=atan2(CollisionPosition(2)-yPositionG3,CollisionPosition(1)-xPositionG3); 
            RotMatrix_0_4=[cos(Theta) -sin(Theta);sin(Theta) cos(Theta)];
end
%............................................................................
%........................................................................
%Absolute Accelerations for G3 and P3 updated from frame 
function RotatedForce = ConvesrsionForceContactPoint(RotMatrix_0_4,Force)
            RotatedForce=RotMatrix_0_4'*Force;
end

    %............................................................................
    %............................................................................
    %Absolute Accelerations for G3 and P3 updated from frame 0
        function RotatedForceToFrame0 = ConvesrsionContactPointFrame0(RotMatrix_0_4,Force)
            RotatedForceToFrame0=RotMatrix_0_4*Force;
        end
    %............................................................................
    %............................................................................
    %Absolute Accelerations for G3 and P3 updated from frame 0
        function ResultantTorque = ResultantTorqueCalc(RotatedForceIndex,RotatedForceThumb)
        global R;
            ResultantTorque=R*RotatedForceIndex+R*RotatedForceThumb;
        end
    %............................................................................
    %............................................................................
    %Absolute Accelerations for G3 and P3 updated from frame 0
        function ResultantForceX=ResultantXForceWithoutFloorFrictionX(IndexForceX,ThumbForceX)
            ResultantForceX=IndexForceX+ThumbForceX;
        end
    %............................................................................
    %............................................................................
    %Absolute Accelerations for G3 and P3 updated from frame 0
        function ResultantForceY=ResultantXForceWithoutFloorFrictionY(IndexForceY,ThumbForceY)
            ResultantForceY=IndexForceY+ThumbForceY;
        end
    %............................................................................
    %............................................................................
    %Absolute Accelerations for G3 and P3 updated from frame 0
        function ForcesInCollision=CollisionConditionFunct(CollisionCondition,FingerForce)
                    if(CollisionCondition==1)
                        ForcesInCollision=FingerForce;
                    else
                        ForcesInCollision=[0;0];
                    end
        end
    %............................................................................
    %............................................................................
    %Absolute Accelerations for G3 and P3 updated from frame 0
        function ForceComponent=ForceVectorAnalysis(GeneralCoordinatesDoubleDot,ForceFingerComp)
        global M;
           if(abs(ForceFingerComp)>=abs(GeneralCoordinatesDoubleDot*M))
               ForceComponent=-ForceFingerComp+GeneralCoordinatesDoubleDot*M;
           else
               ForceComponent=GeneralCoordinatesDoubleDot*M;
           end
        end
    %............................................................................
    %............................................................................
    %Absolute Accelerations for G3 and P3 updated from frame 0
        function ForceReaction=ForceReactionFinger(GeneralCoordinatesDoubleDot,ForceFinger)
           ForceReaction=[0;0];
           ForceComponentIndex=ForceVectorAnalysis(GeneralCoordinatesDoubleDot(1),ForceFinger(1));
           ForceComponentThumb=ForceVectorAnalysis(GeneralCoordinatesDoubleDot(2),ForceFinger(2));
           ForceReaction(1)=ForceComponentIndex;
           ForceReaction(2)=ForceComponentThumb;
           ForceReaction=[ForceReaction(1);ForceReaction(2)];
        end
    %..........................................................................
    %..........................................................................
    %
    function GenCordExt=ForcesCalculator(CollisionIndexForce,CollisionThumbForce,CollisionPosition,...
                                         xPositionG3,yPositionG3)
           RotMatrix_0_4_Index=RotationToContactFrame(CollisionPosition([1 2]),xPositionG3,yPositionG3);
           RotMatrix_0_4_Thumb=RotationToContactFrame(CollisionPosition([3 4]),xPositionG3,yPositionG3);
           RotatedForceIndex = ConvesrsionForceContactPoint(RotMatrix_0_4_Index,CollisionIndexForce);
           RotatedForceThumb = ConvesrsionForceContactPoint(RotMatrix_0_4_Thumb,CollisionThumbForce);
           ResultantTorque = ResultantTorqueCalc(RotatedForceIndex(2),RotatedForceThumb(2));
           ResultantForceX=ResultantXForceWithoutFloorFrictionX(CollisionIndexForce(1),CollisionThumbForce(1));
           ResultantForceY=ResultantXForceWithoutFloorFrictionY(CollisionIndexForce(2),CollisionThumbForce(2));
           GenCordExt=[ResultantForceX,ResultantForceY,ResultantTorque];
    end

== matlab function hybridSysSim/Index/IndexFinger/Index ==
  data: iInitVal input; xDot output; iFa input; iFcSense input; iFeDist input; iO input; rOtoL output; iFcComp output; rOtoLDot output
% Finger Simulink function.
% Represents an underactuated cable driven finger.
% The finger is composed of two phalanges driven by a tendon-pulley
% mechanism. This has methods for calculating the kinematics and
% dynamics of the system.
% Author: Ricardo Garcia Rosas
% Change log:
%%%%%%%%%%%%|%%%%%%%%%%%|%%%%%%%%%%%%%%%%%%%%%%%%%%%%%%%%%%%%%%%%%%%|
% Date      |   Author  | Notes                                     |
% 16/03/23  |   RGR     | Added more comments.                      |
% 16/03/24  |   RGR     | Compute fc and transform to [x,y].        |
% 16/04/06  |   RGR     | Removed force class, using only magnitude.|
% 16/04/09  |   RGR     | Removed classes and opted for functions.  |

function [ xDot, rOtoL, iFcComp, rOtoLDot ] = Finger( iInitVal,iFa,iFcSense,iFeDist,iO )

    % Set initial condition:
    theta = [iInitVal(1); iInitVal(2)];
    thetaDot = [iInitVal(3); iInitVal(4)];
    % Transform forces:
    % Contact force
    fcTN = rotMat(theta(1,1)+theta(2,1))'*iFcSense;
    fcD = fcTN(2,1);
%     if(fcD>0)
%         fcD=0;
%     end
    % Disturbance force
    feTN = rotMat(theta(1,1)+theta(2,1))'*iFeDist;
    feD = feTN(2,1);
    % Set model variables:
    kP = -0.043;
    kD = -0.185;
    dP = -0.01;
    dD = -0.01;
    lP = 0.1;
    lD = 0.1;
    rP = 0.02;
    rD = 0.012;
    aP = 0.1;
    aD = 0.1;
    bP = 0.05;
    bD = 0.05;
    mP = 0.02;
    mD = 0.02;
    theta0 = [pi/10;pi/3];
    IP = mP*(lP^2)/3;
    ID = mD*(lD^2)/12;
    % Set matrices
    K = [kP 0;
         0 kD];
    D = [dP 0;
         0 dD];
    Ja = [rP rD];
    Jc = [aP, 0;
          aD+lP*cos(theta(2,1)),aD];
    Je = [bP, 0;
          bD+lP*cos(theta(2,1)),bD]; 

    % Forward kinematics to link ends and centre of gravity.
    % rOtoL vector from finger origin to link end, one 2D
    % vector for each link.
    % rOtoG vector from finger origin to link center of
    % gravity, one 2D vector for each link.
    rOtoL = zeros(2,2);
    rOtoG = zeros(2,2);
    rOtoL(:,1) = iO + rotMat(theta(1,1))*[lP;0];
    rOtoG(:,1) = iO + rotMat(theta(1,1))*[lP/2;0];
    rOtoL(:,2) = rOtoL(:,2-1) + rotMat(theta(1,1)+theta(2,1))*[lD;0];
    rOtoG(:,2) = rOtoG(:,2-1) + rotMat(theta(1,1)+theta(2,1))*[lD/2;0];
    
    % Dynamics
    rOtoLDot = [-lP*sin(theta(1,1))*thetaDot(1,1)-lD*sin(theta(1,1)+theta(2,1))*(thetaDot(1,1)+thetaDot(2,1));
                -lP*cos(theta(1,1))*thetaDot(1,1)-lD*cos(theta(1,1)+theta(2,1))*(thetaDot(1,1)+thetaDot(2,1))];
    % Compute matrix parameters.
    alpha = IP + ID + (mP*(lP/2)^2) + mD*(lP^2+(lD/2)^2);
    beta = mD*lP*(lD/2);
    delta = ID+mD*(lD/2)^2;
    % Intertia matrix (M)
    M = [alpha+2*beta*cos(theta(2,1)) delta+beta*cos(theta(2,1));
         delta+beta*cos(theta(2,1)) delta];
    % Coriolis and Centrifugal matrix (C)
    C = [-beta*sin(theta(2,1))*thetaDot(2,1) ...
         -beta*sin(theta(2,1))*(thetaDot(1,1)+thetaDot(2,1));
         beta*sin(theta(2,1))*thetaDot(1,1) 0];
    % Torques
    springTau = K*(theta-theta0);
    damperTau = D*thetaDot;
    contactTau = Jc'*[0; fcD];
    distTau = Je'*[0; feD];
    actTau = Ja'*iFa;
    % Compute angular acceleration
    thetaDotDot = inv(M)*(-C*thetaDot + springTau + damperTau + contactTau + distTau + actTau);
    xDot = [thetaDot; thetaDotDot];
    % Compute applied contact force give a static condition. (Kinetostatic)
    % Compute forces normal to proximal and distal links.
    fcComp = (inv(Jc')*(-(springTau+damperTau+distTau+actTau)));
    % Distal normal and tangential (0, no tangential force due to
    % actuation) forces and transform to [x,y] coordinate.
    iFcComp = -rotMat(theta(1,1)+theta(2,1))*[0;fcComp(2,1)];
end
        function rot = rotMat(theta)
            % 2D Z-Rotation matrix on theta.
            % @param theta the angle
            % @return rot the rotation matrix as a 2x2 matrix.
            rot = [cos(theta) -sin(theta);
                   sin(theta) cos(theta)];
        end

== matlab function hybridSysSim/Subsystem/MATLAB Function1 ==
  data: m input; iz output; r input
function iz = fcn(m,r)
%#codegen
    iz=(m*r^2)/2;
end

== matlab function hybridSysSim/Subsystem/MATLAB Function2 ==
  data: m input; g input; fsx output; us input
function fsx = fcn(m,g,us)
%#codegen
    fsx=m*g*us;
end

== matlab function hybridSysSim/Subsystem/MATLAB Function3 ==
  data: m input; fsy output; g input; us input
function fsy = fcn(m,g,us)
%#codegen
    fsy=m*g*us;
end

== matlab function hybridSysSim/Subsystem/MATLAB Function4 ==
  data: m input; fkx output; g input; uk input
function fkx = fcn(m,g,uk)
%#codegen
    fkx=m*g*uk;
end

== matlab function hybridSysSim/Subsystem/MATLAB Function5 ==
  data: m input; fky output; g input; uk input
function fky = fcn(m,g,uk)
%#codegen
    fky=m*g*uk;
end

== matlab function hybridSysSim/Subsystem/MATLAB Function6 ==
  data: urs input; ts output; m input; g input; r input
function ts = fcn(urs,m,g,r)
%#codegen
    ts=(2/3)*urs*r*m*g;
end

== matlab function hybridSysSim/GUI/drawIndex ==
  data: o input; rOtoL input; figNum input
% Plots finger to the default figure. Handled in Simulink.
% Author: Ricardo Garcia Rosas
% Change log:
%%%%%%%%%%%%|%%%%%%%%%%%|%%%%%%%%%%%%%%%%%%%%%%%%%%%%%%%%%%%%%%%%%%%|
% Date      |   Author  | Notes                                     |
% 16/03/23  |   RGR     | Added more comments.                      |
function drawFinger(o,rOtoL,figNum)
    % Plots the finger to the default figure. Handled in Simulink.
    % @param o finger origin position [x,y] (m).
    % @param rOtoL finger vector from its origin to its link
    % ends.
    % @param figNum the figure number for the plot.

    % Call figure
    figure(figNum);
    hold on;
    % Draw Proximal components
    plot([o(1) rOtoL(1,1)],[o(2) rOtoL(2,1)],'LineWidth',8,'Color', 'k');
    plot(o(1),o(2),'ko','MarkerSize',18);
    % Draw Distal components
    plot([rOtoL(1,1) rOtoL(1,2)],[rOtoL(2,1) rOtoL(2,2)],'LineWidth',8,'Color', 'k');
    plot(rOtoL(1,1),rOtoL(2,1),'ko','MarkerSize',18);
    % Draw fingertip
    plot(rOtoL(1,2),rOtoL(2,2),'ko','MarkerSize',8);
    hold off;
    axis([-0.2 0.2 -0.05 0.2]);
end

== matlab function hybridSysSim/Subsystem/MATLAB Function7 ==
  data: urk input; tk output; m input; g input; r input
function tk = fcn(urk,m,g,r)
%#codegen
    tk=(2/3)*urk*r*m*g;
end

== matlab function hybridSysSim/GUI/drawCylinder ==
  data: posG3 input; Position_o_P3 input; R input; figNum input
function DrawCylinder(posG3,Position_o_P3,R,figNum)
%#
    figure(figNum);
    clf;
    hold on
    t=linspace(0,2*pi,360);
    plot(posG3(1,1),posG3(2,1),'r*');
    plot(Position_o_P3(1),Position_o_P3(2),'r*');
    x=posG3(1,1)+R*cos(t);
    y=posG3(2,1)+R*sin(t);
    plot(x,y,'b');
    hold off
    axis([-0.2 0.2 -0.05 0.2]);
end

== matlab function hybridSysSim/Index/Environment/collisionDetection ==
  data: irOtoL input; iCol output; irOtoLDot input; iFcComp input; posG3 input; R input; iColPos output; cRc output
% Handles collision detection between fingertips and Cylinder. 
% Handled in Simulink.
% Author: Ricardo Garcia Rosas
% Change log:
%%%%%%%%%%%%|%%%%%%%%%%%|%%%%%%%%%%%%%%%%%%%%%%%%%%%%%%%%%%%%%%%%%%%|
% Date      |   Author  | Notes                                     |
% 16/04/06  |   RGR     | Created.                                  |
function [iCol,iColPos,cRc] = collisionDetection(irOtoL,irOtoLDot,iFcComp,posG3,R)
    % Handles collision detection between fingertips and Cylinder.
    % Performed by comparing object radius.
    iColPos = zeros(2,1);
    % Get circle radius given object center and fingertip position.
    ri = sqrt((irOtoL(1,2)-posG3(1))^2+(irOtoL(2,2)-posG3(2))^2);
    % Verify calculated radius with object radius to define collision.
    if(ri<=R+0.006)
        iCol = 1;
        iColPos = irOtoL(:,2);
        cRc = (22*0.08*irOtoLDot+iFcComp);
    else
        iCol = 0;
        iColPos = [0;0];
        cRc = [0;0];
    end
    
end
